simulink model "HW2P4c_unstable"  (R2020b)
settings: Solver=VariableStepAuto  StartTime=0.0  StopTime=10.0  RelTol=1e-3
values from neighbouring files (symbols this model uses):
  n = 0 : 120    [HW1.m]
undefined symbols (not defined in the file or in its folder): m
settings Model: Creator=mluser  LastModifiedBy=mluser

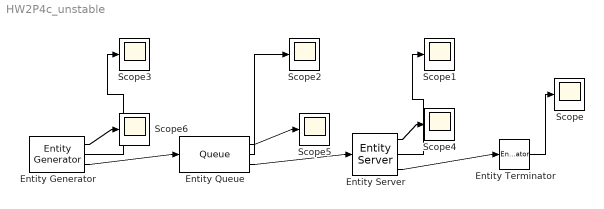
== system HW2P4c_unstable ==
  Entity Generator : EntityGenerator  OutputPortMessageModes=n,n,m  Period=651*10^-6  GenerateAction=|  NumberEntitiesDeparted=on  AverageIntergenerationTime=on  EntityType=Structured  EntityTypeName=Entity
      | persistent rngInit;
      | if isempty(rngInit)
      |     seed = 12345;
      |     rng(seed);
      |     rngInit = true;
      | end
      | 
      | % Pattern: Exponential distribution
      | mu = 1;
      | x = -mu * log(1 - rand());
      settings: OutputPortMap=o0,o2,o3
  Entity Queue : Queue  InputPortMessageModes=m  OutputPortMessageModes=n,n,m  AverageWait=on  AverageQueueLength=on
      settings: OutputPortMap=o2,o3,o5
  Entity Server : EntityServer  InputPortMessageModes=m  OutputPortMessageModes=n,n,m  Capacity=1  ServiceTimeValue=651*10^-6  AverageWait=on  Utilization=on
      settings: OutputPortMap=o4,o5,o9
  Entity Terminator : EntityTerminator  InputPortMessageModes=m  NumberEntitiesArrived=on
      settings: OutputPortMap=o0
  Scope{,1..6} (7 alike) : Scope
  wires:
  Entity Generator/2 -> Scope3/1
  Entity Queue/2 -> Scope2/1
  Entity Queue/1 -> Scope5/1
  Entity Server/1 -> Scope4/1
  Entity Server/2 -> Scope1/1
  Entity Generator/1 -> Scope6/1
  Entity Generator/3 -> Entity Queue/1
  Entity Queue/3 -> Entity Server/1
  Entity Server/3 -> Entity Terminator/1
  Entity Terminator/1 -> Scope/1
